simulink model "lift_stateMachine"  (R2020b)
settings: Solver=VariableStepAuto  StartTime=0.0  StopTime=10.0  RelTol=1e-3
settings Model: Creator=DELL  LastModifiedBy=DELL

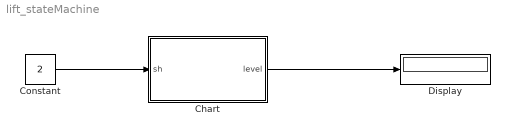
== system lift_stateMachine ==
  Chart : Stateflow chart  TreatAsAtomicUnit=on
  Constant : Constant  Value=2
  Display : Display
  wires:
  Constant/1 -> Chart/1(sh)
  Chart/1(level) -> Display/1

== stateflow chart lift_stateMachine/Chart ==
  state floor4
    entry:
    level=4;
    curr_st=level;
  state floor5
    entry:
    level=5;
    curr_st=level;
  state floor2
    entry:
    level=2;
    curr_st=level;
  state floor3
    entry:
    level=3;
    curr_st=level;
  state floor1
    entry:
    curr_st=1;
    level=1;
  (default) -> floor1
  floor5 -> floor5 [order 2] : [curr_st==5]
  floor3 -> floor4 [order 1] : [curr_st<sh]
  floor4 -> floor5 [order 1] : [curr_st<sh]
  floor2 -> floor3 [order 1] : [curr_st<sh]
  floor1 -> floor2 [order 1] : [curr_st<sh]
  floor1 -> floor1 [order 2] : [curr_st==1]
  floor3 -> floor2 [order 2] : [curr_st>sh]
  floor2 -> floor1 [order 2] : [curr_st>sh]
  floor5 -> floor4 [order 1] : [curr_st>sh]
  floor4 -> floor3 [order 2] : [curr_st>sh]
  data: level output; sh input; curr_st local =0
